simulink model "Demo_PreScanCarSim3D_FMU_cs"  (Simulink 8.6)
settings: Solver=ode5  SolverMode=SingleTasking  StartTime=0.0  StopTime=68  FixedStep=1/1000  RelTol=1e-3
model workspace (MAT data in the model file):
  mbox_table : struct (value not decoded)
  model_closed = 0
  sim_status = 0
PreLoadFcn:
  | mbxruntime.callbacks.PreLoadFcn(bdroot);
  | check_NUTS_defined;
  | 
  | assignin('base',['model_closed_' bdroot],false);
PostLoadFcn:
  | mbxruntime.callbacks.PostLoadFcn(bdroot);
InitFcn:
  | mbxruntime.callbacks.InitFcn(bdroot);
StartFcn:
  | mbxruntime.callbacks.StartFcn(bdroot);
StopFcn:
  | mbxruntime.callbacks.StopFcn(bdroot);
undefined symbols (not defined in the file or in its folder): DiscIntNeverNeededParam, mbxruntime, tabledata, warningInitialVelocity, x0, x_ini_VRML, y_ini_VRML, z_ini_VRML
libraries: PreScanSimulinkLibrary x15, simulink_extras x8, simulink x5, PreScanCarSimLibrary x1, fmu_cs_lib x1
(part 1 of 11)
CloseFcn:
  | mbxruntime.callbacks.CloseFcn(bdroot);
  | evalin('base',['clear model_closed_' bdroot]);
settings Model: Creator=PRESCAN  LastModifiedBy=woudstm
settings OptimizationCC: BooleanDataType=off  InitFltsAndDblsToZero=on
settings DebuggingCC: SaveWithParameterizedLinksMsg=none  SignalResolutionControl=TryResolveAllWithWarning  SolverPrmCheckMsg=none  MultiTaskDSMMsg=warning  MultiTaskCondExecSysMsg=none  FcnCallInpInsideContextMsg=UseLocalSettings
settings ModelReferenceCC: UpdateModelReferenceTargets=IfOutOfDate
settings SFSimCC: SimParseCustomCode=off
settings SFSimCC: SimCustomHeaderCode=|
  | #include "prescan.h"
  | #include "prescan_platform.h"
settings GRTTargetCC: TargetFcnLib=ansi_tfl_tmw.mat

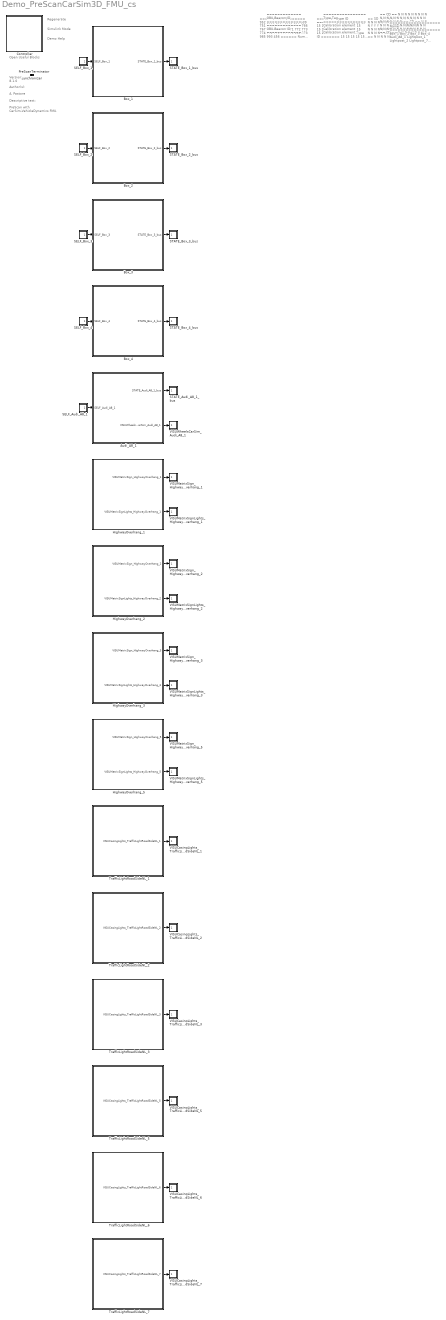
== system Demo_PreScanCarSim3D_FMU_cs ==
  note: Regenerate
  note: Simulink Mode
  note: Open Useful Blocks
  note: 8.1.0
  note: Version:
  note: Author(s):
  note: A. Pastore
  note: Descriptive text:
  note: PreScan with
      | CarSim-VehicleDynamics FMU.
  note: Demo Help
  note: ======
      | Num ID
      | ======
      | 952
      | 1033
      | 1034
      | 1035
      | 296
      | 639
      | 751
      | 761
      | 762
      | 763
      | 764
      | 765
      | 766
      | 767
      | 768
      | 769
      | 770
      | 771
      | 772
      | 773
      | 774
      | 775
      | 776
      | 777
      | 778
      | 115
      | 973
      | 985
      | 993
      | 456
      | ======
      | Num ID
      | ======
      | 457
      | 458
      | 459
      | 460
      | 461
      | 462
      | 463
      | 464
      | 465
      | 560
      | 561
      | 499
      | 641
      | 642
      | 644
      | 645
      | 646
      | 639
      | 751
      | 761
      | 762
      | 763
      | 764
      | 765
      | 766
      | 767
      | 768
      | 769
      | 770
      | 771
      | ======
      | Num ID
      | ======
      | 772
      | 773
      | 774
      | 775
      | 776
      | 777
      | 778
      | 115
      | 973
      | 985
      | 993
      | 456
      | 457
      | 458
      | 459
      | 460
      | 461
      | 462
      | 463
      | 464
      | 465
      | 560
      | 561
      | 499
      | 641
      | 642
      | 644
      | 645
      | 646
      | 647
      | ======
      | Num ID
      | ======
      | 908
      | 909
      | 910
      | 911
      | 928
      | 929
      | 930
      | 931
  note: =============
      | OBU-Beacon ID
      | =============
      |
      |
      |
      |
      |
      |
      |
      |
      |
      |
      |
      |
      |
      |
      |
      |
      |
      |
      |
      |
      |
      |
      |
      |
      |
      |
      |
      |
      |
      |
      | =============
      | OBU-Beacon ID
      | =============
      |
      |
      |
      |
      |
      |
      |
      |
      |
      |
      |
      |
      |
      |
      |
      |
      |
      |
      |
      |
      |
      |
      |
      |
      |
      |
      |
      |
      |
      |
      | =============
      | OBU-Beacon ID
      | =============
      |
      |
      |
      |
      |
      |
      |
      |
      |
      |
      |
      |
      |
      |
      |
      |
      |
      |
      |
      |
      |
      |
      |
      |
      |
      |
      |
      |
      |
      |
      | =============
      | OBU-Beacon ID
      | =============
  note: =======
      | Type ID
      | =======
      | 5
      | 5
      | 5
      | 5
      | 1
      | 15
      | 15
      | 15
      | 15
      | 15
      | 15
      | 15
      | 15
      | 15
      | 15
      | 15
      | 15
      | 15
      | 15
      | 15
      | 15
      | 15
      | 15
      | 15
      | 15
      | 15
      | 15
      | 15
      | 15
      | 15
      | =======
      | Type ID
      | =======
      | 15
      | 15
      | 15
      | 15
      | 15
      | 15
      | 15
      | 15
      | 15
      | 15
      | 15
      | 15
      | 15
      | 15
      | 15
      | 15
      | 15
      | 15
      | 15
      | 15
      | 15
      | 15
      | 15
      | 15
      | 15
      | 15
      | 15
      | 15
      | 15
      | 15
      | =======
      | Type ID
      | =======
      | 15
      | 15
      | 15
      | 15
      | 15
      | 15
      | 15
      | 15
      | 15
      | 15
      | 15
      | 15
      | 15
      | 15
      | 15
      | 15
      | 15
      | 15
      | 15
      | 15
      | 15
      | 15
      | 15
      | 15
      | 15
      | 15
      | 15
      | 15
      | 15
      | 15
      | =======
      | Type ID
      | =======
      | 15
      | 15
      | 15
      | 15
      | 15
      | 15
      | 15
      | 15
  note: ================
      | Type Tag
      | ================
      | Calibration element
      | Calibration element
      | Calibration element
      | Calibration element
      | Car
      | Animated traffic sign
      | Animated traffic sign
      | Animated traffic sign
      | Animated traffic sign
      | Animated traffic sign
      | Animated traffic sign
      | Animated traffic sign
      | Animated traffic sign
      | Animated traffic sign
      | Animated traffic sign
      | Animated traffic sign
      | Animated traffic sign
      | Animated traffic sign
      | Animated traffic sign
      | Animated traffic sign
      | Animated traffic sign
      | Animated traffic sign
      | Animated traffic sign
      | Animated traffic sign
      | Animated traffic sign
      | Animated traffic sign
      | Animated traffic sign
      | Animated traffic sign
      | Animated traffic sign
      | Animated traffic sign
      | ================
      | Type Tag
      | ================
      | Animated traffic sign
      | Animated traffic sign
      | Animated traffic sign
      | Animated traffic sign
      | Animated traffic sign
      | Animated traffic sign
      | Animated traffic sign
      | Animated traffic sign
      | Animated traffic sign
      | Animated traffic sign
      | Animated traffic sign
      | Animated traffic sign
      | Animated traffic sign
      | Animated traffic sign
      | Animated traffic sign
      | Animated traffic sign
      | Animated traffic sign
      | Animated traffic sign
      | Animated traffic sign
      | Animated traffic sign
      | Animated traffic sign
      | Animated traffic sign
      | Animated traffic sign
      | Animated traffic sign
      | Animated traffic sign
      | Animated traffic sign
      | Animated traffic sign
      | Animated traffic sign
      | Animated traffic sign
      | Animated traffic sign
      | ================
      | Type Tag
      | ================
      | Animated traffic sign
      | Animated traffic sign
      | Animated traffic sign
      | Animated traffic sign
      | Animated traffic sign
      | Animated traffic sign
      | Animated traffic sign
      | Animated traffic sign
      | Animated traffic sign
      | Animated traffic sign
      | Animated traffic sign
      | Animated traffic sign
      | Animated traffic sign
      | Animated traffic sign
      | Animated traffic sign
      | Animated traffic sign
      | Animated traffic sign
      | Animated traffic sign
      | Animated traffic sign
      | Animated traffic sign
      | Animated traffic sign
      | Animated traffic sign
      | Animated traffic sign
      | Animated traffic sign
      | Animated traffic sign
      | Animated traffic sign
      | Animated traffic sign
      | Animated traffic sign
      | Animated traffic sign
      | Animated traffic sign
      | ================
      | Type Tag
      | ================
      | Animated traffic sign
      | Animated traffic sign
      | Animated traffic sign
      | Animated traffic sign
      | Animated traffic sign
      | Animated traffic sign
      | Animated traffic sign
      | Animated traffic sign
  note: ==
      | SD
      | ==
      | Y
      | Y
      | Y
      | Y
      | Y
      | N
      | N
      | N
      | N
      | N
      | N
      | N
      | N
      | N
      | N
      | N
      | N
      | N
      | N
      | N
      | N
      | N
      | N
      | N
      | N
      | Y
      | Y
      | Y
      | Y
      | N
      | ==
      | SD
      | ==
      | N
      | N
      | N
      | N
      | N
      | N
      | N
      | N
      | N
      | N
      | N
      | Y
      | Y
      | Y
      | Y
      | Y
      | Y
      | N
      | N
      | N
      | N
      | N
      | N
      | N
      | N
      | N
      | N
      | N
      | N
      | N
      | ==
      | SD
      | ==
      | N
      | N
      | N
      | N
      | N
      | N
      | N
      | Y
      | Y
      | Y
      | Y
      | N
      | N
      | N
      | N
      | N
      | N
      | N
      | N
      | N
      | N
      | N
      | N
      | Y
      | Y
      | Y
      | Y
      | Y
      | Y
      | Y
      | ==
      | SD
      | ==
      | Y
      | Y
      | Y
      | Y
      | Y
      | Y
      | Y
      | Y
  note: ==
      | CD
      | ==
      | N
      | N
      | N
      | N
      | N
      | N
      | N
      | N
      | N
      | N
      | N
      | N
      | N
      | N
      | N
      | N
      | N
      | N
      | N
      | N
      | N
      | N
      | N
      | N
      | N
      | N
      | N
      | N
      | N
      | N
      | ==
      | CD
      | ==
      | N
      | N
      | N
      | N
      | N
      | N
      | N
      | N
      | N
      | N
      | N
      | N
      | N
      | N
      | N
      | N
      | N
      | N
      | N
      | N
      | N
      | N
      | N
      | N
      | N
      | N
      | N
      | N
      | N
      | N
      | ==
      | CD
      | ==
      | N
      | N
      | N
      | N
      | N
      | N
      | N
      | N
      | N
      | N
      | N
      | N
      | N
      | N
      | N
      | N
      | N
      | N
      | N
      | N
      | N
      | N
      | N
      | N
      | N
      | N
      | N
      | N
      | N
      | N
      | ==
      | CD
      | ==
      | N
      | N
      | N
      | N
      | N
      | N
      | N
      | N
  note: ===================
      | Name
      | ===================
      | Box_1
      | Box_2
      | Box_3
      | Box_4
      | Audi_A8_1
      | Lightpost_1
      | Lightpost_2
      | Lightpost_7
      | Lightpost_8
      | Lightpost_9
      | Lightpost_10
      | Lightpost_11
      | Lightpost_12
      | Lightpost_13
      | Lightpost_14
      | Lightpost_15
      | Lightpost_16
      | Lightpost_17
      | Lightpost_18
      | Lightpost_19
      | Lightpost_20
      | Lightpost_21
      | Lightpost_22
      | Lightpost_23
      | Lightpost_24
      | HighwayOverhang_1
      | HighwayOverhang_2
      | HighwayOverhang_3
      | HighwayOverhang_5
      | Lightpost_25
      | ===================
      | Name
      | ===================
      | Lightpost_26
      | Lightpost_27
      | Lightpost_28
      | Lightpost_29
      | Lightpost_30
      | Lightpost_31
      | Lightpost_32
      | Lightpost_33
      | Lightpost_34
      | Lightpost_35
      | Lightpost_36
      | TrafficLightRoadSideNL_1
      | TrafficLightRoadSideNL_2
      | TrafficLightRoadSideNL_3
      | TrafficLightRoadSideNL_5
      | TrafficLightRoadSideNL_6
      | TrafficLightRoadSideNL_7
      | Lightpost_1
      | Lightpost_2
      | Lightpost_7
      | Lightpost_8
      | Lightpost_9
      | Lightpost_10
      | Lightpost_11
      | Lightpost_12
      | Lightpost_13
      | Lightpost_14
      | Lightpost_15
      | Lightpost_16
      | Lightpost_17
      | ===================
      | Name
      | ===================
      | Lightpost_18
      | Lightpost_19
      | Lightpost_20
      | Lightpost_21
      | Lightpost_22
      | Lightpost_23
      | Lightpost_24
      | HighwayOverhang_1
      | HighwayOverhang_2
      | HighwayOverhang_3
      | HighwayOverhang_5
      | Lightpost_25
      | Lightpost_26
      | Lightpost_27
      | Lightpost_28
      | Lightpost_29
      | Lightpost_30
      | Lightpost_31
      | Lightpost_32
      | Lightpost_33
      | Lightpost_34
      | Lightpost_35
      | Lightpost_36
      | TrafficLightRoadSideNL_1
      | TrafficLightRoadSideNL_2
      | TrafficLightRoadSideNL_3
      | TrafficLightRoadSideNL_5
      | TrafficLightRoadSideNL_6
      | TrafficLightRoadSideNL_7
      | InformationBoard_2
      | ===================
      | Name
      | ===================
      | InformationBoard_5
      | InformationBoard_6
      | InformationBoard_7
      | InformationBoard_8
      | InformationBoard_25
      | InformationBoard_26
      | InformationBoard_27
      | InformationBoard_28
  Audi_A8_1 : Subsystem  Tag=WorldObjectSubSystem  InitFcn=UniqueId = '3037';  Variant=on  OverrideUsingVariant=on
      mask init:
      | imagePath=which('Audi_A8.jpg');
      settings: OpenFcn=open_system([gcb '/ENABLED'])
      mask Display: image(imread(imagePath));color('white');text(0,0,' ID=296\n')
  Box_1 : Subsystem  Tag=WorldObjectSubSystem  InitFcn=UniqueId = '2076';  Variant=on  OverrideUsingVariant=on
      mask init:
      | imagePath=which('Box.jpg');
      settings: OpenFcn=open_system([gcb '/ENABLED'])
      mask Display: image(imread(imagePath));color('white');text(0,0,' ID=952\n')
  Box_2 : Subsystem  Tag=WorldObjectSubSystem  InitFcn=UniqueId = '2077';  Variant=on  OverrideUsingVariant=on
      mask init:
      | imagePath=which('Box.jpg');
      settings: OpenFcn=open_system([gcb '/ENABLED'])
      mask Display: image(imread(imagePath));color('white');text(0,0,' ID=1033\n')
  Box_3 : Subsystem  Tag=WorldObjectSubSystem  InitFcn=UniqueId = '2078';  Variant=on  OverrideUsingVariant=on
      mask init:
      | imagePath=which('Box.jpg');
      settings: OpenFcn=open_system([gcb '/ENABLED'])
      mask Display: image(imread(imagePath));color('white');text(0,0,' ID=1034\n')
  Box_4 : Subsystem  Tag=WorldObjectSubSystem  InitFcn=UniqueId = '2079';  Variant=on  OverrideUsingVariant=on
      mask init:
      | imagePath=which('Box.jpg');
      settings: OpenFcn=open_system([gcb '/ENABLED'])
      mask Display: image(imread(imagePath));color('white');text(0,0,' ID=1035\n')
  Controller : Subsystem  Description=0BD42F5D76B3CBB80C42962BC42B91E5A71A983F04A5119EDD9D2B7D55C4E295  Priority=-1  LoadFcn=load PreScanControllerData  mask(PreScan Simulation Controller){prescanversion='8.1.0', ModelReferencing=off, TimeStep=50/1000, ControlMode=0, PreScanExecutionMode=on, ControllerCount=0, ControllerIndex=0, ControllerOptions=''}
      mask prompts: prescanversion "PreScan Version"; ModelReferencing "Use Model Referencing"; TimeStep "Upload Period [s]"; ControlMode "Control Mode"; PreScanExecutionMode "Execution Mode"; ControllerCount "Controller Count"; ControllerIndex "Controller Index"; ControllerOptions "Controller Options"
      mask help:
      | Please do not remove this block from the compilation sheet,
      | as it connects the model to the PreScan environment.
      mask init:
      | model = bdroot(gcb);
      | ExperimentFile = mbxruntime.findExperimentFile(model);
      | 
      | [d1, d2, d3, prescandata] = prescan_Settings();
      | ModelDepo = fullfile(prescandata,'ModelDepo'); 
      | 
      | RTmode = 0;
      | actors = find_system(model,'SearchDepth', 1,'LookUnderMasks', 'all','Tag','WorldObjectSubSystem');
      | for ii=1:length(actors)
      |     actormode = get_param(actors{ii},'OverrideUsingVariant');
      |     if strcmpi(actormode,'off')
      |         RTmode = 1;
      |     end
      | end
      | 
      | SimulationMode = get_param(bdroot,'SimulationMode');
      | if strcmp(SimulationMode, 'rapid-accelerator')
      |     SimulationMode = 'external';
      | end
      | TargetName = get_param(bdroot,'SystemTargetFile');
      settings: ModelCloseFcn=assignin('base',['model_closed_' bdroot],true);
      mask Help: eval('openHelp(812)')
      mask Display: image(imread('prescanlogo.ico'))
  HighwayOverhang_1 : Subsystem  Tag=WorldObjectSubSystem  InitFcn=UniqueId = '1876';  Variant=on  OverrideUsingVariant=on
      mask init:
      | imagePath=which('HighwayOverhang.jpg');
      settings: OpenFcn=open_system([gcb '/ENABLED'])
      mask Display: image(imread(imagePath));color('white');text(0,0,' ID=115\n')
  HighwayOverhang_2 : Subsystem  Tag=WorldObjectSubSystem  InitFcn=UniqueId = '1877';  Variant=on  OverrideUsingVariant=on
      mask init:
      | imagePath=which('HighwayOverhang.jpg');
      settings: OpenFcn=open_system([gcb '/ENABLED'])
      mask Display: image(imread(imagePath));color('white');text(0,0,' ID=973\n')
  HighwayOverhang_3 : Subsystem  Tag=WorldObjectSubSystem  InitFcn=UniqueId = '1890';  Variant=on  OverrideUsingVariant=on
      mask init:
      | imagePath=which('HighwayOverhang.jpg');
      settings: OpenFcn=open_system([gcb '/ENABLED'])
      mask Display: image(imread(imagePath));color('white');text(0,0,' ID=985\n')
  HighwayOverhang_5 : Subsystem  Tag=WorldObjectSubSystem  InitFcn=UniqueId = '1909';  Variant=on  OverrideUsingVariant=on
      mask init:
      | imagePath=which('HighwayOverhang.jpg');
      settings: OpenFcn=open_system([gcb '/ENABLED'])
      mask Display: image(imread(imagePath));color('white');text(0,0,' ID=993\n')
  PreScanTerminator : Subsystem  Tag=PreScanTerminator  Priority=999  LoadFcn=load PrescanTerminatorData  mask(PreScan Simulation Terminator){TimeStep=50/1000}
      mask prompts: TimeStep "Upload Period [s]"
      mask help:
      | Please do not remove this block from the compilation sheet as it
      | connects the model to the PreScan environment.
      mask Help: eval('openHelp(812)')
      mask Display: image(imread('prescanlogo.ico'))
  SELF_Audi_A8_1 : Subsystem  Tag=sensor/SelfPort  Priority=3  LoadFcn=load('PreScanSelfSensorData.mat')  Variant=on  OverrideUsingVariant=on  mask(PreScan Source Block: SELF){}
      mask help:
      | The SELF port shows (state) information of the actor itself. The outputs are position in the experiment's axis system and the GPS coordinates, and the object's absolute velocity and compass heading.
      |
      | For more information, please click Help.
      settings: OpenFcn=open_system([gcb '/ENABLED/Sensor'],'mask')
      mask Help: eval('openHelp(462)')
      mask Display: image(imread('GPS.png'))
  SELF_Box_1 : Subsystem  Tag=sensor/SelfPort  Priority=3  LoadFcn=load('PreScanSelfSensorData.mat')  Variant=on  OverrideUsingVariant=on  mask(PreScan Source Block: SELF){}
      mask help:
      | The SELF port shows (state) information of the actor itself. The outputs are position in the experiment's axis system and the GPS coordinates, and the object's absolute velocity and compass heading.
      |
      | For more information, please click Help.
      settings: OpenFcn=open_system([gcb '/ENABLED/Sensor'],'mask')
      mask Help: eval('openHelp(462)')
      mask Display: image(imread('GPS.png'))
  SELF_Box_2 : Subsystem  Tag=sensor/SelfPort  Priority=3  LoadFcn=load('PreScanSelfSensorData.mat')  Variant=on  OverrideUsingVariant=on  mask(PreScan Source Block: SELF){}
      mask help:
      | The SELF port shows (state) information of the actor itself. The outputs are position in the experiment's axis system and the GPS coordinates, and the object's absolute velocity and compass heading.
      |
      | For more information, please click Help.
      settings: OpenFcn=open_system([gcb '/ENABLED/Sensor'],'mask')
      mask Help: eval('openHelp(462)')
      mask Display: image(imread('GPS.png'))
  SELF_Box_3 : Subsystem  Tag=sensor/SelfPort  Priority=3  LoadFcn=load('PreScanSelfSensorData.mat')  Variant=on  OverrideUsingVariant=on  mask(PreScan Source Block: SELF){}
      mask help:
      | The SELF port shows (state) information of the actor itself. The outputs are position in the experiment's axis system and the GPS coordinates, and the object's absolute velocity and compass heading.
      |
      | For more information, please click Help.
      settings: OpenFcn=open_system([gcb '/ENABLED/Sensor'],'mask')
      mask Help: eval('openHelp(462)')
      mask Display: image(imread('GPS.png'))
  SELF_Box_4 : Subsystem  Tag=sensor/SelfPort  Priority=3  LoadFcn=load('PreScanSelfSensorData.mat')  Variant=on  OverrideUsingVariant=on  mask(PreScan Source Block: SELF){}
      mask help:
      | The SELF port shows (state) information of the actor itself. The outputs are position in the experiment's axis system and the GPS coordinates, and the object's absolute velocity and compass heading.
      |
      | For more information, please click Help.
      settings: OpenFcn=open_system([gcb '/ENABLED/Sensor'],'mask')
      mask Help: eval('openHelp(462)')
      mask Display: image(imread('GPS.png'))
  STATE_Audi_A8_1_bus : Subsystem  Tag=actuator/StatePort  Priority=0  LoadFcn=load('PreScanStateActuatorData.mat')  Variant=on  OverrideUsingVariant=on  mask(PreScan Sink Block: State){}
      mask help:
      | The Actor State contains a vector signal of size (9x1), containing the following signals:
      |
      | -  Position    	(x,y,z)             	[m]
      | -  Velocity    	(vx,vy,vz)         	[m/s]
      | -  Angles       	(Roll, Pitch, Yaw)	[rad]
      |
      | The Actor state is defined in the global axis system.
      | The state is superponed on the Initial position defined in the GUI.
      |
      | For more information, please click Help.
      settings: OpenFcn=open_system([gcb '/ENABLED/Actuator'],'mask')
      mask Help: eval('openHelp(222)')
      mask Display: image(imread('State.png'))
  STATE_Box_1_bus : Subsystem  Tag=actuator/StatePort  Priority=0  LoadFcn=load('PreScanStateActuatorData.mat')  Variant=on  OverrideUsingVariant=on  mask(PreScan Sink Block: State){}
      mask help:
      | The Actor State contains a vector signal of size (9x1), containing the following signals:
      |
      | -  Position    	(x,y,z)             	[m]
      | -  Velocity    	(vx,vy,vz)         	[m/s]
      | -  Angles       	(Roll, Pitch, Yaw)	[rad]
      |
      | The Actor state is defined in the global axis system.
      | The state is superponed on the Initial position defined in the GUI.
      |
      | For more information, please click Help.
      settings: OpenFcn=open_system([gcb '/ENABLED/Actuator'],'mask')
      mask Help: eval('openHelp(222)')
      mask Display: image(imread('State.png'))
  STATE_Box_2_bus : Subsystem  Tag=actuator/StatePort  Priority=0  LoadFcn=load('PreScanStateActuatorData.mat')  Variant=on  OverrideUsingVariant=on  mask(PreScan Sink Block: State){}
      mask help:
      | The Actor State contains a vector signal of size (9x1), containing the following signals:
      |
      | -  Position    	(x,y,z)             	[m]
      | -  Velocity    	(vx,vy,vz)         	[m/s]
      | -  Angles       	(Roll, Pitch, Yaw)	[rad]
      |
      | The Actor state is defined in the global axis system.
      | The state is superponed on the Initial position defined in the GUI.
      |
      | For more information, please click Help.
      settings: OpenFcn=open_system([gcb '/ENABLED/Actuator'],'mask')
      mask Help: eval('openHelp(222)')
      mask Display: image(imread('State.png'))
  STATE_Box_3_bus : Subsystem  Tag=actuator/StatePort  Priority=0  LoadFcn=load('PreScanStateActuatorData.mat')  Variant=on  OverrideUsingVariant=on  mask(PreScan Sink Block: State){}
      mask help:
      | The Actor State contains a vector signal of size (9x1), containing the following signals:
      |
      | -  Position    	(x,y,z)             	[m]
      | -  Velocity    	(vx,vy,vz)         	[m/s]
      | -  Angles       	(Roll, Pitch, Yaw)	[rad]
      |
      | The Actor state is defined in the global axis system.
      | The state is superponed on the Initial position defined in the GUI.
      |
      | For more information, please click Help.
      settings: OpenFcn=open_system([gcb '/ENABLED/Actuator'],'mask')
      mask Help: eval('openHelp(222)')
      mask Display: image(imread('State.png'))
  STATE_Box_4_bus : Subsystem  Tag=actuator/StatePort  Priority=0  LoadFcn=load('PreScanStateActuatorData.mat')  Variant=on  OverrideUsingVariant=on  mask(PreScan Sink Block: State){}
      mask help:
      | The Actor State contains a vector signal of size (9x1), containing the following signals:
      |
      | -  Position    	(x,y,z)             	[m]
      | -  Velocity    	(vx,vy,vz)         	[m/s]
      | -  Angles       	(Roll, Pitch, Yaw)	[rad]
      |
      | The Actor state is defined in the global axis system.
      | The state is superponed on the Initial position defined in the GUI.
      |
      | For more information, please click Help.
      settings: OpenFcn=open_system([gcb '/ENABLED/Actuator'],'mask')
      mask Help: eval('openHelp(222)')
      mask Display: image(imread('State.png'))
  Synchronizer : Subsystem  Tag=PreScanSynchronizer  Priority=1  LoadFcn=load PrescanSynchronizeData  mask(PreScan Simulation Core Block){TimeStep=50/1000}
      mask prompts: TimeStep "Timestep [s]"
      mask help:
      | Please do not remove this block from the PreScan compilation sheet,
      | as it contains essential configuration parameters for a PreScan simulation.
      settings: DeleteFcn=PreScanBlockDeleteFcn;
      mask Display: image(imread('prescanlogo.ico'))
  TrafficLightRoadSideNL_1 : Subsystem  Tag=WorldObjectSubSystem  InitFcn=UniqueId = '2553';  Variant=on  OverrideUsingVariant=on
      mask init:
      | imagePath=which('TrafficLightRoadSideNL.jpg');
      settings: OpenFcn=open_system([gcb '/ENABLED'])
      mask Display: image(imread(imagePath));color('white');text(0,0,' ID=499\n')
  TrafficLightRoadSideNL_2 : Subsystem  Tag=WorldObjectSubSystem  InitFcn=UniqueId = '2554';  Variant=on  OverrideUsingVariant=on
      mask init:
      | imagePath=which('TrafficLightRoadSideNL.jpg');
      settings: OpenFcn=open_system([gcb '/ENABLED'])
      mask Display: image(imread(imagePath));color('white');text(0,0,' ID=641\n')
  TrafficLightRoadSideNL_3 : Subsystem  Tag=WorldObjectSubSystem  InitFcn=UniqueId = '2555';  Variant=on  OverrideUsingVariant=on
      mask init:
      | imagePath=which('TrafficLightRoadSideNL.jpg');
      settings: OpenFcn=open_system([gcb '/ENABLED'])
      mask Display: image(imread(imagePath));color('white');text(0,0,' ID=642\n')
  TrafficLightRoadSideNL_5 : Subsystem  Tag=WorldObjectSubSystem  InitFcn=UniqueId = '2557';  Variant=on  OverrideUsingVariant=on
      mask init:
      | imagePath=which('TrafficLightRoadSideNL.jpg');
      settings: OpenFcn=open_system([gcb '/ENABLED'])
      mask Display: image(imread(imagePath));color('white');text(0,0,' ID=644\n')
  TrafficLightRoadSideNL_6 : Subsystem  Tag=WorldObjectSubSystem  InitFcn=UniqueId = '2558';  Variant=on  OverrideUsingVariant=on
      mask init:
      | imagePath=which('TrafficLightRoadSideNL.jpg');
      settings: OpenFcn=open_system([gcb '/ENABLED'])
      mask Display: image(imread(imagePath));color('white');text(0,0,' ID=645\n')
  TrafficLightRoadSideNL_7 : Subsystem  Tag=WorldObjectSubSystem  InitFcn=UniqueId = '2559';  Variant=on  OverrideUsingVariant=on
      mask init:
      | imagePath=which('TrafficLightRoadSideNL.jpg');
      settings: OpenFcn=open_system([gcb '/ENABLED'])
      mask Display: image(imread(imagePath));color('white');text(0,0,' ID=646\n')
  VISUCasingLights_TrafficLightRoadSideNL_1 : Subsystem  Tag=actuator/VisuCasingLights  Priority=0  Variant=on  OverrideUsingVariant=on  mask(PreScan Sink Block: VisuTrafficLight){UniqueID=2553, ColorsObjectQuery=, Colors=[]}
      mask prompts: UniqueID "Parent Unique Identifier"; ColorsObjectQuery "Query for Color Object"; Colors "Matrix of colors"
      mask help:
      | The VisuTrafficLight block provides a way to animate traffic lights: switch on and off individual lights.
      |
      | For more information, please click Help.
      settings: OpenFcn=open_system([gcb '/ENABLED/Actuator'],'mask')
      mask Help: eval('openHelp(731)')
      mask Display: image(imread('TrafficLightCasing.png'))
  VISUCasingLights_TrafficLightRoadSideNL_2 : Subsystem  Tag=actuator/VisuCasingLights  Priority=0  Variant=on  OverrideUsingVariant=on  mask(PreScan Sink Block: VisuTrafficLight){UniqueID=2554, ColorsObjectQuery=, Colors=[]}
      mask prompts: UniqueID "Parent Unique Identifier"; ColorsObjectQuery "Query for Color Object"; Colors "Matrix of colors"
      mask help:
      | The VisuTrafficLight block provides a way to animate traffic lights: switch on and off individual lights.
      |
      | For more information, please click Help.
      settings: OpenFcn=open_system([gcb '/ENABLED/Actuator'],'mask')
      mask Help: eval('openHelp(731)')
      mask Display: image(imread('TrafficLightCasing.png'))
  VISUCasingLights_TrafficLightRoadSideNL_3 : Subsystem  Tag=actuator/VisuCasingLights  Priority=0  Variant=on  OverrideUsingVariant=on  mask(PreScan Sink Block: VisuTrafficLight){UniqueID=2555, ColorsObjectQuery=, Colors=[]}
      mask prompts: UniqueID "Parent Unique Identifier"; ColorsObjectQuery "Query for Color Object"; Colors "Matrix of colors"
      mask help:
      | The VisuTrafficLight block provides a way to animate traffic lights: switch on and off individual lights.
      |
      | For more information, please click Help.
      settings: OpenFcn=open_system([gcb '/ENABLED/Actuator'],'mask')
      mask Help: eval('openHelp(731)')
      mask Display: image(imread('TrafficLightCasing.png'))
  VISUCasingLights_TrafficLightRoadSideNL_5 : Subsystem  Tag=actuator/VisuCasingLights  Priority=0  Variant=on  OverrideUsingVariant=on  mask(PreScan Sink Block: VisuTrafficLight){UniqueID=2557, ColorsObjectQuery=, Colors=[]}
      mask prompts: UniqueID "Parent Unique Identifier"; ColorsObjectQuery "Query for Color Object"; Colors "Matrix of colors"
      mask help:
      | The VisuTrafficLight block provides a way to animate traffic lights: switch on and off individual lights.
      |
      | For more information, please click Help.
      settings: OpenFcn=open_system([gcb '/ENABLED/Actuator'],'mask')
      mask Help: eval('openHelp(731)')
      mask Display: image(imread('TrafficLightCasing.png'))
  VISUCasingLights_TrafficLightRoadSideNL_6 : Subsystem  Tag=actuator/VisuCasingLights  Priority=0  Variant=on  OverrideUsingVariant=on  mask(PreScan Sink Block: VisuTrafficLight){UniqueID=2558, ColorsObjectQuery=, Colors=[]}
      mask prompts: UniqueID "Parent Unique Identifier"; ColorsObjectQuery "Query for Color Object"; Colors "Matrix of colors"
      mask help:
      | The VisuTrafficLight block provides a way to animate traffic lights: switch on and off individual lights.
      |
      | For more information, please click Help.
      settings: OpenFcn=open_system([gcb '/ENABLED/Actuator'],'mask')
      mask Help: eval('openHelp(731)')
      mask Display: image(imread('TrafficLightCasing.png'))
  VISUCasingLights_TrafficLightRoadSideNL_7 : Subsystem  Tag=actuator/VisuCasingLights  Priority=0  Variant=on  OverrideUsingVariant=on  mask(PreScan Sink Block: VisuTrafficLight){UniqueID=2559, ColorsObjectQuery=, Colors=[]}
      mask prompts: UniqueID "Parent Unique Identifier"; ColorsObjectQuery "Query for Color Object"; Colors "Matrix of colors"
      mask help:
      | The VisuTrafficLight block provides a way to animate traffic lights: switch on and off individual lights.
      |
      | For more information, please click Help.
      settings: OpenFcn=open_system([gcb '/ENABLED/Actuator'],'mask')
      mask Help: eval('openHelp(731)')
      mask Display: image(imread('TrafficLightCasing.png'))
  VISUMatrixSignLights_HighwayOverhang_1 : Subsystem  Tag=actuator/VisuMatrixSignLights  Priority=0  Variant=on  OverrideUsingVariant=on  mask(PreScan Sink Block: VisuMatrixSignLights){UniqueID=1876, ColorsObjectQuery=, Colors=[]}
      mask prompts: UniqueID "Parent Unique Identifier"; ColorsObjectQuery "Query for Color Object"; Colors "Matrix of colors"
      mask help:
      | The VisuMatrixSignLights block provides a way to switch the lights on the matrix sign board on or off
      |
      | For more information, please click Help.
      settings: OpenFcn=open_system([gcb '/ENABLED/Actuator'],'mask')
      mask Help: eval('openHelp(732)')
      mask Display: image(imread('RearLight.png'))
  VISUMatrixSignLights_HighwayOverhang_2 : Subsystem  Tag=actuator/VisuMatrixSignLights  Priority=0  Variant=on  OverrideUsingVariant=on  mask(PreScan Sink Block: VisuMatrixSignLights){UniqueID=1877, ColorsObjectQuery=, Colors=[]}
      mask prompts: UniqueID "Parent Unique Identifier"; ColorsObjectQuery "Query for Color Object"; Colors "Matrix of colors"
      mask help:
      | The VisuMatrixSignLights block provides a way to switch the lights on the matrix sign board on or off
      |
      | For more information, please click Help.
      settings: OpenFcn=open_system([gcb '/ENABLED/Actuator'],'mask')
      mask Help: eval('openHelp(732)')
      mask Display: image(imread('RearLight.png'))
  VISUMatrixSignLights_HighwayOverhang_3 : Subsystem  Tag=actuator/VisuMatrixSignLights  Priority=0  Variant=on  OverrideUsingVariant=on  mask(PreScan Sink Block: VisuMatrixSignLights){UniqueID=1890, ColorsObjectQuery=, Colors=[]}
      mask prompts: UniqueID "Parent Unique Identifier"; ColorsObjectQuery "Query for Color Object"; Colors "Matrix of colors"
      mask help:
      | The VisuMatrixSignLights block provides a way to switch the lights on the matrix sign board on or off
      |
      | For more information, please click Help.
      settings: OpenFcn=open_system([gcb '/ENABLED/Actuator'],'mask')
      mask Help: eval('openHelp(732)')
      mask Display: image(imread('RearLight.png'))
  VISUMatrixSignLights_HighwayOverhang_5 : Subsystem  Tag=actuator/VisuMatrixSignLights  Priority=0  Variant=on  OverrideUsingVariant=on  mask(PreScan Sink Block: VisuMatrixSignLights){UniqueID=1909, ColorsObjectQuery=, Colors=[]}
      mask prompts: UniqueID "Parent Unique Identifier"; ColorsObjectQuery "Query for Color Object"; Colors "Matrix of colors"
      mask help:
      | The VisuMatrixSignLights block provides a way to switch the lights on the matrix sign board on or off
      |
      | For more information, please click Help.
      settings: OpenFcn=open_system([gcb '/ENABLED/Actuator'],'mask')
      mask Help: eval('openHelp(732)')
      mask Display: image(imread('RearLight.png'))
  VISUMatrixSign_HighwayOverhang_1 : Subsystem  Tag=actuator/VisuMatrixSign  Priority=0  Variant=on  OverrideUsingVariant=on  mask(PreScan Sink Block: VisuMatrixSign){UniqueID=1876, ResourceList={'3' 'InformationSign\MatrixSign_Empty.png' '4' 'InformationSign\MatrixSign_End.png' '5' 'InformationSign\MatrixSign_GreenArrow.png' '6' 'InformationSign\MatrixSign_RedCross.png' '7' 'InformationSign\MatrixSign_Speed_50.png' '8' 'InformationSign\MatrixSign_Speed_70.png' '9' 'InformationSign\MatrixSign_Speed_90.png' '10' 'InformationSign\MatrixSign_Speed_120.png' '11' 'InformationSign\MatrixSign_Speed_130.png' '12' 'InformationSign\information.png' '13' 'InformationSign\TASS-international-logo.bmp' }, PivotName=}
      mask prompts: UniqueID "Parent Unique Identifier (auto-generated)"; ResourceList "Resource List (auto-generated)"; PivotName "Name of pivot (auto-generated)"
      mask help:
      | The VisuMatrixSign block provides a way to adapt the texture of the plates connected to an overhang, based on Resource IDs of the texture files.
      |
      | For more information, please click Help.
      settings: OpenFcn=open_system([gcb '/ENABLED/Actuator'],'mask')
      mask Help: eval('openHelp(733)')
      mask Display: image(imread('HighwaySpeedMatrix.png'))
  VISUMatrixSign_HighwayOverhang_2 : Subsystem  Tag=actuator/VisuMatrixSign  Priority=0  Variant=on  OverrideUsingVariant=on  mask(PreScan Sink Block: VisuMatrixSign){UniqueID=1877, ResourceList={'3' 'InformationSign\MatrixSign_Empty.png' '4' 'InformationSign\MatrixSign_End.png' '5' 'InformationSign\MatrixSign_GreenArrow.png' '6' 'InformationSign\MatrixSign_RedCross.png' '7' 'InformationSign\MatrixSign_Speed_50.png' '8' 'InformationSign\MatrixSign_Speed_70.png' '9' 'InformationSign\MatrixSign_Speed_90.png' '10' 'InformationSign\MatrixSign_Speed_120.png' '11' 'InformationSign\MatrixSign_Speed_130.png' '12' 'InformationSign\information.png' '13' 'InformationSign\TASS-international-logo.bmp' }, PivotName=}
      mask prompts: UniqueID "Parent Unique Identifier (auto-generated)"; ResourceList "Resource List (auto-generated)"; PivotName "Name of pivot (auto-generated)"
      mask help:
      | The VisuMatrixSign block provides a way to adapt the texture of the plates connected to an overhang, based on Resource IDs of the texture files.
      |
      | For more information, please click Help.
      settings: OpenFcn=open_system([gcb '/ENABLED/Actuator'],'mask')
      mask Help: eval('openHelp(733)')
      mask Display: image(imread('HighwaySpeedMatrix.png'))
  VISUMatrixSign_HighwayOverhang_3 : Subsystem  Tag=actuator/VisuMatrixSign  Priority=0  Variant=on  OverrideUsingVariant=on  mask(PreScan Sink Block: VisuMatrixSign){UniqueID=1890, ResourceList={'3' 'InformationSign\MatrixSign_Empty.png' '4' 'InformationSign\MatrixSign_End.png' '5' 'InformationSign\MatrixSign_GreenArrow.png' '6' 'InformationSign\MatrixSign_RedCross.png' '7' 'InformationSign\MatrixSign_Speed_50.png' '8' 'InformationSign\MatrixSign_Speed_70.png' '9' 'InformationSign\MatrixSign_Speed_90.png' '10' 'InformationSign\MatrixSign_Speed_120.png' '11' 'InformationSign\MatrixSign_Speed_130.png' '12' 'InformationSign\information.png' '13' 'InformationSign\TASS-international-logo.bmp' }, PivotName=}
      mask prompts: UniqueID "Parent Unique Identifier (auto-generated)"; ResourceList "Resource List (auto-generated)"; PivotName "Name of pivot (auto-generated)"
      mask help:
      | The VisuMatrixSign block provides a way to adapt the texture of the plates connected to an overhang, based on Resource IDs of the texture files.
      |
      | For more information, please click Help.
      settings: OpenFcn=open_system([gcb '/ENABLED/Actuator'],'mask')
      mask Help: eval('openHelp(733)')
      mask Display: image(imread('HighwaySpeedMatrix.png'))
  VISUMatrixSign_HighwayOverhang_5 : Subsystem  Tag=actuator/VisuMatrixSign  Priority=0  Variant=on  OverrideUsingVariant=on  mask(PreScan Sink Block: VisuMatrixSign){UniqueID=1909, ResourceList={'3' 'InformationSign\MatrixSign_Empty.png' '4' 'InformationSign\MatrixSign_End.png' '5' 'InformationSign\MatrixSign_GreenArrow.png' '6' 'InformationSign\MatrixSign_RedCross.png' '7' 'InformationSign\MatrixSign_Speed_50.png' '8' 'InformationSign\MatrixSign_Speed_70.png' '9' 'InformationSign\MatrixSign_Speed_90.png' '10' 'InformationSign\MatrixSign_Speed_120.png' '11' 'InformationSign\MatrixSign_Speed_130.png' '12' 'InformationSign\information.png' '13' 'InformationSign\TASS-international-logo.bmp' }, PivotName=}
      mask prompts: UniqueID "Parent Unique Identifier (auto-generated)"; ResourceList "Resource List (auto-generated)"; PivotName "Name of pivot (auto-generated)"
      mask help:
      | The VisuMatrixSign block provides a way to adapt the texture of the plates connected to an overhang, based on Resource IDs of the texture files.
      |
      | For more information, please click Help.
      settings: OpenFcn=open_system([gcb '/ENABLED/Actuator'],'mask')
      mask Help: eval('openHelp(733)')
      mask Display: image(imread('HighwaySpeedMatrix.png'))
  VISUWheelsCarSim_Audi_A8_1 : Subsystem  Tag=Actuator  Priority=0  LoadFcn=load('PrescanAxisAngleData');load('PrescanXYZData')  Variant=on  OverrideUsingVariant=on  mask(PreScan User Interface: VisuWheels){}
      mask help:
      | The VisuWheels block provides a way to animate the wheels of a vehicle, with steering, rotation (because of velocity) and z-displacement.
      |
      | For more information, please click Help.
      settings: OpenFcn=open_system([gcb '/ENABLED/Actuator'],'mask')
      mask Help: eval('openHelp(223)')
      mask Display: image(imread('wheel.png'))
  wires:
  Box_1/1(STATE_Box_1_bus) -> STATE_Box_1_bus/1(STATE_Box_1_bus)
  SELF_Box_1/1(SELF_Box_1) -> Box_1/1(SELF_Box_1)
  Box_2/1(STATE_Box_2_bus) -> STATE_Box_2_bus/1(STATE_Box_2_bus)
  SELF_Box_2/1(SELF_Box_2) -> Box_2/1(SELF_Box_2)
  Box_3/1(STATE_Box_3_bus) -> STATE_Box_3_bus/1(STATE_Box_3_bus)
  SELF_Box_3/1(SELF_Box_3) -> Box_3/1(SELF_Box_3)
  Box_4/1(STATE_Box_4_bus) -> STATE_Box_4_bus/1(STATE_Box_4_bus)
  SELF_Box_4/1(SELF_Box_4) -> Box_4/1(SELF_Box_4)
  Audi_A8_1/1(STATE_Audi_A8_1_bus) -> STATE_Audi_A8_1_bus/1(STATE_Audi_A8_1_bus)
  SELF_Audi_A8_1/1(SELF_Audi_A8_1) -> Audi_A8_1/1(SELF_Audi_A8_1)
  Audi_A8_1/2(VISUWheelsCarSim_Audi_A8_1) -> VISUWheelsCarSim_Audi_A8_1/1(VISUWheelsCarSim_Audi_A8_1)
  HighwayOverhang_1/1(VISUMatrixSign_HighwayOverhang_1) -> VISUMatrixSign_HighwayOverhang_1/1(VISUMatrixSign_HighwayOverhang_1)
  HighwayOverhang_1/2(VISUMatrixSignLights_HighwayOverhang_1) -> VISUMatrixSignLights_HighwayOverhang_1/1(VISUMatrixSignLights_HighwayOverhang_1)
  HighwayOverhang_2/1(VISUMatrixSign_HighwayOverhang_2) -> VISUMatrixSign_HighwayOverhang_2/1(VISUMatrixSign_HighwayOverhang_2)
  HighwayOverhang_2/2(VISUMatrixSignLights_HighwayOverhang_2) -> VISUMatrixSignLights_HighwayOverhang_2/1(VISUMatrixSignLights_HighwayOverhang_2)
  HighwayOverhang_3/1(VISUMatrixSign_HighwayOverhang_3) -> VISUMatrixSign_HighwayOverhang_3/1(VISUMatrixSign_HighwayOverhang_3)
  HighwayOverhang_3/2(VISUMatrixSignLights_HighwayOverhang_3) -> VISUMatrixSignLights_HighwayOverhang_3/1(VISUMatrixSignLights_HighwayOverhang_3)
  HighwayOverhang_5/1(VISUMatrixSign_HighwayOverhang_5) -> VISUMatrixSign_HighwayOverhang_5/1(VISUMatrixSign_HighwayOverhang_5)
  HighwayOverhang_5/2(VISUMatrixSignLights_HighwayOverhang_5) -> VISUMatrixSignLights_HighwayOverhang_5/1(VISUMatrixSignLights_HighwayOverhang_5)
  TrafficLightRoadSideNL_1/1(VISUCasingLights_TrafficLightRoadSideNL_1) -> VISUCasingLights_TrafficLightRoadSideNL_1/1(VISUCasingLights_TrafficLightRoadSideNL_1)
  TrafficLightRoadSideNL_2/1(VISUCasingLights_TrafficLightRoadSideNL_2) -> VISUCasingLights_TrafficLightRoadSideNL_2/1(VISUCasingLights_TrafficLightRoadSideNL_2)
  TrafficLightRoadSideNL_3/1(VISUCasingLights_TrafficLightRoadSideNL_3) -> VISUCasingLights_TrafficLightRoadSideNL_3/1(VISUCasingLights_TrafficLightRoadSideNL_3)
  TrafficLightRoadSideNL_5/1(VISUCasingLights_TrafficLightRoadSideNL_5) -> VISUCasingLights_TrafficLightRoadSideNL_5/1(VISUCasingLights_TrafficLightRoadSideNL_5)
  TrafficLightRoadSideNL_6/1(VISUCasingLights_TrafficLightRoadSideNL_6) -> VISUCasingLights_TrafficLightRoadSideNL_6/1(VISUCasingLights_TrafficLightRoadSideNL_6)
  TrafficLightRoadSideNL_7/1(VISUCasingLights_TrafficLightRoadSideNL_7) -> VISUCasingLights_TrafficLightRoadSideNL_7/1(VISUCasingLights_TrafficLightRoadSideNL_7)

== system Demo_PreScanCarSim3D_FMU_cs/Audi_A8_1 ==
  SELF_Audi_A8_1 : Inport  Tag=inport/SelfPort  OutDataTypeStr=Bus: PRESCAN_SELFSENSORDATA  PortDimensions=1  SampleTime=50/1000  BusOutputAsStruct=on
  DISABLED : Subsystem  VariantControl=off
  ENABLED : Subsystem  VariantControl=on
  STATE_Audi_A8_1_bus : Outport  Tag=outport/StatePort  OutDataTypeStr=Bus: PRESCAN_STATEACTUATORDATA  PortDimensions=1  SampleTime=50/1000
  VISUWheelsCarSim_Audi_A8_1 : Outport  Tag=outport/VisuWheels  Port=2  SampleTime=50/1000

== system Demo_PreScanCarSim3D_FMU_cs/Box_1 ==
  SELF_Box_1 : Inport  Tag=inport/SelfPort  OutDataTypeStr=Bus: PRESCAN_SELFSENSORDATA  PortDimensions=1  SampleTime=50/1000  BusOutputAsStruct=on
  DISABLED : Subsystem  VariantControl=off
  ENABLED : Subsystem  VariantControl=on
  STATE_Box_1_bus : Outport  Tag=outport/StatePort  OutDataTypeStr=Bus: PRESCAN_STATEACTUATORDATA  PortDimensions=1  SampleTime=50/1000

== system Demo_PreScanCarSim3D_FMU_cs/Box_2 ==
  SELF_Box_2 : Inport  Tag=inport/SelfPort  OutDataTypeStr=Bus: PRESCAN_SELFSENSORDATA  PortDimensions=1  SampleTime=50/1000  BusOutputAsStruct=on
  DISABLED : Subsystem  VariantControl=off
  ENABLED : Subsystem  VariantControl=on
  STATE_Box_2_bus : Outport  Tag=outport/StatePort  OutDataTypeStr=Bus: PRESCAN_STATEACTUATORDATA  PortDimensions=1  SampleTime=50/1000

== system Demo_PreScanCarSim3D_FMU_cs/Box_3 ==
  SELF_Box_3 : Inport  Tag=inport/SelfPort  OutDataTypeStr=Bus: PRESCAN_SELFSENSORDATA  PortDimensions=1  SampleTime=50/1000  BusOutputAsStruct=on
  DISABLED : Subsystem  VariantControl=off
  ENABLED : Subsystem  VariantControl=on
  STATE_Box_3_bus : Outport  Tag=outport/StatePort  OutDataTypeStr=Bus: PRESCAN_STATEACTUATORDATA  PortDimensions=1  SampleTime=50/1000

== system Demo_PreScanCarSim3D_FMU_cs/Box_4 ==
  SELF_Box_4 : Inport  Tag=inport/SelfPort  OutDataTypeStr=Bus: PRESCAN_SELFSENSORDATA  PortDimensions=1  SampleTime=50/1000  BusOutputAsStruct=on
  DISABLED : Subsystem  VariantControl=off
  ENABLED : Subsystem  VariantControl=on
  STATE_Box_4_bus : Outport  Tag=outport/StatePort  OutDataTypeStr=Bus: PRESCAN_STATEACTUATORDATA  PortDimensions=1  SampleTime=50/1000

== system Demo_PreScanCarSim3D_FMU_cs/Controller ==
  Terminator : Terminator
  sfun_Controller : S-Function  FunctionName=sfun_Controller  Parameters=SParameter1, SParameter2, SParameter3, SParameter4, SParameter5, SParameter6, SParameter7, SParameter8, SParameter9, SParameter10, SampleTime  SFunctionDeploymentMode=off  EnableBusSupport=off  mask(Legacy Function){SFunctionSpec=void prescan_outputFcn(void** work1, PRESCAN_CONTROLLERDATA y1[1]), SParameter1=uint8([ExperimentFile 0]), SParameter2=uint8([ModelDepo 0]), SParameter3=uint8([ControllerOptions 0]), SParameter4=RTmode, SParameter5=PreScanExecutionMode, SParameter6=ControlMode, SParameter7=ControllerCount, SParameter8=ControllerIndex, SParameter9=uint8([SimulationMode 0]), SParameter10=uint8([TargetName 0]), SampleTime=TimeStep, ShowSpec=on}
      mask prompts: SParameter1 "P1:"; SParameter2 "P2:"; SParameter3 "P3:"; SParameter4 "P4:"; SParameter5 "P5:"; SParameter6 "P6:"; SParameter7 "P7:"; SParameter8 "P8:"; SParameter9 "P9:"; SParameter10 "P10:"; SampleTime "Sample time (-1 for inherited):"; ShowSpec "Display function specification"
      mask help:
      | This block allows you to call the legacy functions specified by the following Legacy Code Tool definition:
      | def.SFunctionName = 'sfun_Controller';
      | def.OutputFcnSpec = 'void prescan_outputFcn(void** work1, PRESCAN_CONTROLLERDATA y1[1])';
      | def.StartFcnSpec = 'void prescan_startFcn(void ** work1, uint8 p1[], uint8 p2[], uint8 p3[], double p4, double p5, double p6, double p7, double p8, uint8 p9[], uint8 p10[])';
      | def.TerminateFcnSpec = 'void prescan_terminateFcn(void** work1)';
      | def.HeaderFiles = {'prescan_controller_data.h', 'prescan_SFunLibrary.h', 'prescan_LogHandler.h', 'prescan_CreateLogHandler.h', 'prescan_ErrorHandler.h', 'prescan_CreateErrorHandler.h', 'prescan_modify.h', 'ModuleDLL.h'};
      | def.SourceFiles = {'prescan_MexLogHandler.cpp', 'prescan_SimStructErrorHandler.cpp', 'prescan_LogHandler.cpp', 'prescan_ErrorHandler.cpp', 'prescan_Modify.cpp'};
      | def.HostLibFiles = {'sensorinterfaced.lib'};
      | def.TargetLibFiles = {'sensorinterfaced.so'};
      | def.IncPaths = {'.', 'C:\projects\prescan\rt_vislibrary\vis\..\pimp\include\sensors\InterfaceRTW'};
      | def.SrcPaths = {'C:\projects\prescan\rt_vislibrary\vis\..\pimp\include\sensors\InterfaceRTW', 'C:\projects\prescan\rt_vislibrary\vis\..\pimp\include\sensors\InterfaceRTW\ccurrt'};
      | def.LibPaths = {'C:\\projects\\prescan\\vislibrary_build\lib'};
      | def.SampleTime = 'parameterized';
      mask Help: <p>This block was generated automatically by the Legacy Code Tool. For detailed help on this tool, call<a href="matlab:legacy_code('help')"> legacy_code('help')</a>.</p>
      mask Callback ShowSpec:
      | if strcmp(get_param(gcbh, 'ShowSpec'), 'on')
      |   set_param(gcbh, 'MaskDisplay', sprintf('fprintf(''%s'');', get_param(gcbh, 'SFunctionSpec')));
      | else
      |   set_param(gcbh, 'MaskDisplay', sprintf('fprintf(''%s'');', get_param(gcbh, 'FunctionName')));
      | end
      mask Display: fprintf('void prescan_outputFcn(void** work1, PRESCAN_CONTROLLERDATA y1[1])');
  wires:
  sfun_Controller/1 -> Terminator/1

== system Demo_PreScanCarSim3D_FMU_cs/HighwayOverhang_1 ==
  DISABLED : Subsystem  VariantControl=off
  ENABLED : Subsystem  VariantControl=on
  VISUMatrixSign_HighwayOverhang_1 : Outport  Tag=outport/VisuMatrixSign  SampleTime=50/1000
  VISUMatrixSignLights_HighwayOverhang_1 : Outport  Tag=outport/VisuMatrixSignLights  Port=2  SampleTime=50/1000

== system Demo_PreScanCarSim3D_FMU_cs/HighwayOverhang_2 ==
  DISABLED : Subsystem  VariantControl=off
  ENABLED : Subsystem  VariantControl=on
  VISUMatrixSign_HighwayOverhang_2 : Outport  Tag=outport/VisuMatrixSign  SampleTime=50/1000
  VISUMatrixSignLights_HighwayOverhang_2 : Outport  Tag=outport/VisuMatrixSignLights  Port=2  SampleTime=50/1000

== system Demo_PreScanCarSim3D_FMU_cs/HighwayOverhang_3 ==
  DISABLED : Subsystem  VariantControl=off
  ENABLED : Subsystem  VariantControl=on
  VISUMatrixSign_HighwayOverhang_3 : Outport  Tag=outport/VisuMatrixSign  SampleTime=50/1000
  VISUMatrixSignLights_HighwayOverhang_3 : Outport  Tag=outport/VisuMatrixSignLights  Port=2  SampleTime=50/1000

== system Demo_PreScanCarSim3D_FMU_cs/HighwayOverhang_5 ==
  DISABLED : Subsystem  VariantControl=off
  ENABLED : Subsystem  VariantControl=on
  VISUMatrixSign_HighwayOverhang_5 : Outport  Tag=outport/VisuMatrixSign  SampleTime=50/1000
  VISUMatrixSignLights_HighwayOverhang_5 : Outport  Tag=outport/VisuMatrixSignLights  Port=2  SampleTime=50/1000

== system Demo_PreScanCarSim3D_FMU_cs/PreScanTerminator ==
  Terminator : Terminator
  sfun_Terminator : S-Function  FunctionName=sfun_Terminator  Parameters=SampleTime  SFunctionDeploymentMode=off  EnableBusSupport=off  mask(Legacy Function){SFunctionSpec=void prescan_terminator_outputFcn(void ** work1, PRESCAN_TERMINATORDATA y1[1]), SampleTime=TimeStep, ShowSpec=on}
      mask prompts: SampleTime "Sample time (-1 for inherited):"; ShowSpec "Display function specification"
      mask help:
      | This block allows you to call the legacy functions specified by the following Legacy Code Tool definition:
      | def.SFunctionName = 'sfun_Terminator';
      | def.OutputFcnSpec = 'void prescan_terminator_outputFcn(void ** work1, PRESCAN_TERMINATORDATA y1[1])';
      | def.StartFcnSpec = 'void prescan_terminator_startFcn(void ** work1)';
      | def.TerminateFcnSpec = 'void prescan_terminator_terminateFcn(void ** work1)';
      | def.HeaderFiles = {'prescan_terminator_data.h'};
      | def.HostLibFiles = {'sensorinterfaced.lib'};
      | def.IncPaths = {'src', 'C:\prescandev\vislibrary\vis\..\pimp\include\sensors\InterfaceRTW'};
      | def.SrcPaths = {'src'};
      | def.LibPaths = {'C:\\prescandev\\vislibrary_build\lib'};
      | def.SampleTime = 'parameterized';
      | def.Options.language = 'C++';
      mask Help: <p>This block was generated automatically by the Legacy Code Tool. For detailed help on this tool, call<a href="matlab:legacy_code('help')"> legacy_code('help')</a>.</p>
      mask Callback ShowSpec:
      | if strcmp(get_param(gcbh, 'ShowSpec'), 'on')
      |   set_param(gcbh, 'MaskDisplay', sprintf('fprintf(''%s'');', get_param(gcbh, 'SFunctionSpec')));
      | else
      |   set_param(gcbh, 'MaskDisplay', sprintf('fprintf(''%s'');', get_param(gcbh, 'FunctionName')));
      | end
      mask Display: fprintf('void prescan_terminator_outputFcn(void ** work1, PRESCAN_TERMINATORDATA y1[1])');
  wires:
  sfun_Terminator/1 -> Terminator/1

== system Demo_PreScanCarSim3D_FMU_cs/SELF_Audi_A8_1 ==
  DISABLED : Subsystem  VariantControl=off
  ENABLED : Subsystem  VariantControl=on
  SELF_Audi_A8_1 : Outport  Tag=outport/SelfPort  OutDataTypeStr=Bus: PRESCAN_SELFSENSORDATA  PortDimensions=1  SampleTime=50/1000

== system Demo_PreScanCarSim3D_FMU_cs/SELF_Box_1 ==
  DISABLED : Subsystem  VariantControl=off
  ENABLED : Subsystem  VariantControl=on
  SELF_Box_1 : Outport  Tag=outport/SelfPort  OutDataTypeStr=Bus: PRESCAN_SELFSENSORDATA  PortDimensions=1  SampleTime=50/1000

== system Demo_PreScanCarSim3D_FMU_cs/SELF_Box_2 ==
  DISABLED : Subsystem  VariantControl=off
  ENABLED : Subsystem  VariantControl=on
  SELF_Box_2 : Outport  Tag=outport/SelfPort  OutDataTypeStr=Bus: PRESCAN_SELFSENSORDATA  PortDimensions=1  SampleTime=50/1000

== system Demo_PreScanCarSim3D_FMU_cs/SELF_Box_3 ==
  DISABLED : Subsystem  VariantControl=off
  ENABLED : Subsystem  VariantControl=on
  SELF_Box_3 : Outport  Tag=outport/SelfPort  OutDataTypeStr=Bus: PRESCAN_SELFSENSORDATA  PortDimensions=1  SampleTime=50/1000

== system Demo_PreScanCarSim3D_FMU_cs/SELF_Box_4 ==
  DISABLED : Subsystem  VariantControl=off
  ENABLED : Subsystem  VariantControl=on
  SELF_Box_4 : Outport  Tag=outport/SelfPort  OutDataTypeStr=Bus: PRESCAN_SELFSENSORDATA  PortDimensions=1  SampleTime=50/1000

== system Demo_PreScanCarSim3D_FMU_cs/STATE_Audi_A8_1_bus ==
  STATE_Audi_A8_1_bus : Inport  Tag=inport/StatePort  OutDataTypeStr=Bus: PRESCAN_STATEACTUATORDATA  PortDimensions=1  SampleTime=50/1000  BusOutputAsStruct=on
  DISABLED : Subsystem  VariantControl=off
  ENABLED : Subsystem  VariantControl=on

== system Demo_PreScanCarSim3D_FMU_cs/STATE_Box_1_bus ==
  STATE_Box_1_bus : Inport  Tag=inport/StatePort  OutDataTypeStr=Bus: PRESCAN_STATEACTUATORDATA  PortDimensions=1  SampleTime=50/1000  BusOutputAsStruct=on
  DISABLED : Subsystem  VariantControl=off
  ENABLED : Subsystem  VariantControl=on

== system Demo_PreScanCarSim3D_FMU_cs/STATE_Box_2_bus ==
  STATE_Box_2_bus : Inport  Tag=inport/StatePort  OutDataTypeStr=Bus: PRESCAN_STATEACTUATORDATA  PortDimensions=1  SampleTime=50/1000  BusOutputAsStruct=on
  DISABLED : Subsystem  VariantControl=off
  ENABLED : Subsystem  VariantControl=on

== system Demo_PreScanCarSim3D_FMU_cs/STATE_Box_3_bus ==
  STATE_Box_3_bus : Inport  Tag=inport/StatePort  OutDataTypeStr=Bus: PRESCAN_STATEACTUATORDATA  PortDimensions=1  SampleTime=50/1000  BusOutputAsStruct=on
  DISABLED : Subsystem  VariantControl=off
  ENABLED : Subsystem  VariantControl=on

== system Demo_PreScanCarSim3D_FMU_cs/STATE_Box_4_bus ==
  STATE_Box_4_bus : Inport  Tag=inport/StatePort  OutDataTypeStr=Bus: PRESCAN_STATEACTUATORDATA  PortDimensions=1  SampleTime=50/1000  BusOutputAsStruct=on
  DISABLED : Subsystem  VariantControl=off
  ENABLED : Subsystem  VariantControl=on

== system Demo_PreScanCarSim3D_FMU_cs/Synchronizer ==
  Bus Selector1 : BusSelector  OutputSignals=FederateStopped
  Stop Simulation : Stop
  sfun_Synchronizer : S-Function  FunctionName=sfun_Synchronizer  Parameters=SampleTime  SFunctionDeploymentMode=off  EnableBusSupport=off  mask(Legacy Function){SFunctionSpec=void prescan_synchronizer_outputFcn(void ** work1, PRESCAN_SYNCHRONIZEDATA y1[1]), SampleTime=TimeStep, ShowSpec=on}
      mask prompts: SampleTime "Sample time (-1 for inherited):"; ShowSpec "Display function specification"
      mask help:
      | This block allows you to call the legacy functions specified by the following Legacy Code Tool definition:
      | def.SFunctionName = 'sfun_Synchronizer';
      | def.OutputFcnSpec = 'void prescan_synchronizer_outputFcn(void ** work1, PRESCAN_SYNCHRONIZEDATA y1[1])';
      | def.StartFcnSpec = 'void prescan_synchronizer_startFcn(void ** work1)';
      | def.TerminateFcnSpec = 'void prescan_synchronizer_terminateFcn(void ** work1)';
      | def.HeaderFiles = {'prescan_synchronizer_data.h'};
      | def.HostLibFiles = {'sensorinterfaced.lib'};
      | def.IncPaths = {'src', 'C:\prescandev\vislibrary\vis\..\pimp\include\sensors\InterfaceRTW'};
      | def.SrcPaths = {'src'};
      | def.LibPaths = {'C:\\prescandev\\vislibrary_build\lib'};
      | def.SampleTime = 'parameterized';
      | def.Options.language = 'C++';
      mask Help: <p>This block was generated automatically by the Legacy Code Tool. For detailed help on this tool, call<a href="matlab:legacy_code('help')"> legacy_code('help')</a>.</p>
      mask Callback ShowSpec:
      | if strcmp(get_param(gcbh, 'ShowSpec'), 'on')
      |   set_param(gcbh, 'MaskDisplay', sprintf('fprintf(''%s'');', get_param(gcbh, 'SFunctionSpec')));
      | else
      |   set_param(gcbh, 'MaskDisplay', sprintf('fprintf(''%s'');', get_param(gcbh, 'FunctionName')));
      | end
      mask Display: fprintf('void prescan_synchronizer_outputFcn(void ** work1, PRESCAN_SYNCHRONIZEDATA y1[1])');
  wires:
  Bus Selector1/1 -> Stop Simulation/1  "<FederateStopped>"
  sfun_Synchronizer/1 -> Bus Selector1/1

== system Demo_PreScanCarSim3D_FMU_cs/TrafficLightRoadSideNL_1 ==
  DISABLED : Subsystem  VariantControl=off
  ENABLED : Subsystem  VariantControl=on
  VISUCasingLights_TrafficLightRoadSideNL_1 : Outport  Tag=outport/VisuCasingLights  SampleTime=50/1000
